simulink model "Big_system"  (R2025b)
settings: Solver=ode8  StartTime=0.0  StopTime=60*80  FixedStep=1  RelTol=1e-3
model workspace (MAT data in the model file):
  Sig = Simulink.Signal
  Sig.Dimensions = -1
  Sig.DimensionsMode = 'auto'
  Sig.Complexity = 'auto'
  Sig.SampleTime = -1
  Sig.SamplingMode = 'auto'
  Sig.DataType = 'auto'
settings Model: Creator=Soere  LastModifiedBy=klump
settings DebuggingCC: UnderSpecifiedDimensionMsg=warning

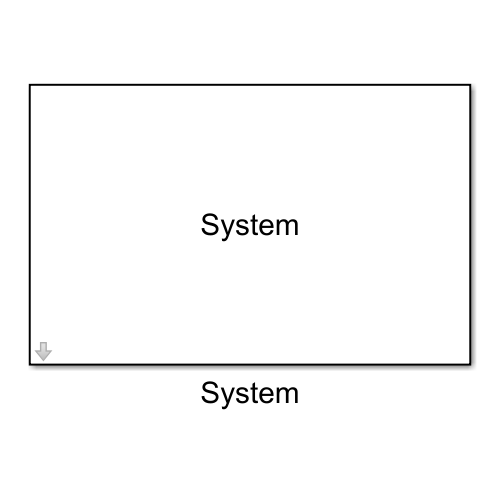
[thumbnail: Simulink's stored preview of the top-level diagram]
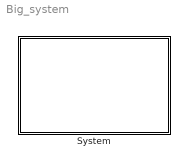
== system Big_system ==
  System : Subsystem  mask{RainSmallStart=(60*20)/4 * 0, RainSmall=5/5, RainSmallDur=60*20, RainBig=20/5, RainBigDur=(60*20)/4, ProcessingRate=9, flip_order=off, EnableBurst_1=on, EnableBurst_4=off, EnableBurst_2=off, EnableBurst_5=on, EnableBurst_3=off, EnableBurst_6=off}
      mask prompts: RainSmallStart "Start of rain:"; RainSmall "Normal rainfall (liters/minute):"; RainSmallDur "Normal Rainfall Duration:"; RainBig "Cloudburst (liters/minute):"; RainBigDur "Cloudburst duration (sec):"; ProcessingRate "Processing rate:"; flip_order "Flip order"; EnableBurst_1 "Enable cloud burst 1"; EnableBurst_4 "Enable cloud burst 4"; EnableBurst_2 "Enable cloud burst 2"; EnableBurst_5 "Enable cloud burst 5"; EnableBurst_3 "Enable cloud burst 3"; EnableBurst_6 "Enable cloud burst 6"
      mask TypeOptions flip_order: Final/flip_order | Subsystem 1/flip_order | Subsystem 1/flip_order_2 | Subsystem 2/flip_order | Subsystem 2/flip_order_2 | Subsystem 3/flip_order | Subsystem 4/flip_order | Subsystem 4/flip_order_2 | Subsystem 5/flip_order | Subsystem 6/flip_order | Subsystem 6/flip_order_2
      mask TypeOptions EnableBurst_1: Subsystem 1/EnableBurst
      mask TypeOptions EnableBurst_4: Subsystem 4/EnableBurst
      mask TypeOptions EnableBurst_2: Subsystem 2/EnableBurst
      mask TypeOptions EnableBurst_5: Subsystem 5/EnableBurst
      mask TypeOptions EnableBurst_3: Subsystem 3/EnableBurst
      mask TypeOptions EnableBurst_6: Final/EnableBurst | Subsystem 6/EnableBurst
      mask DialogControl Container3 Prompt: Enable cloudbursts:
      mask Display: disp('System');

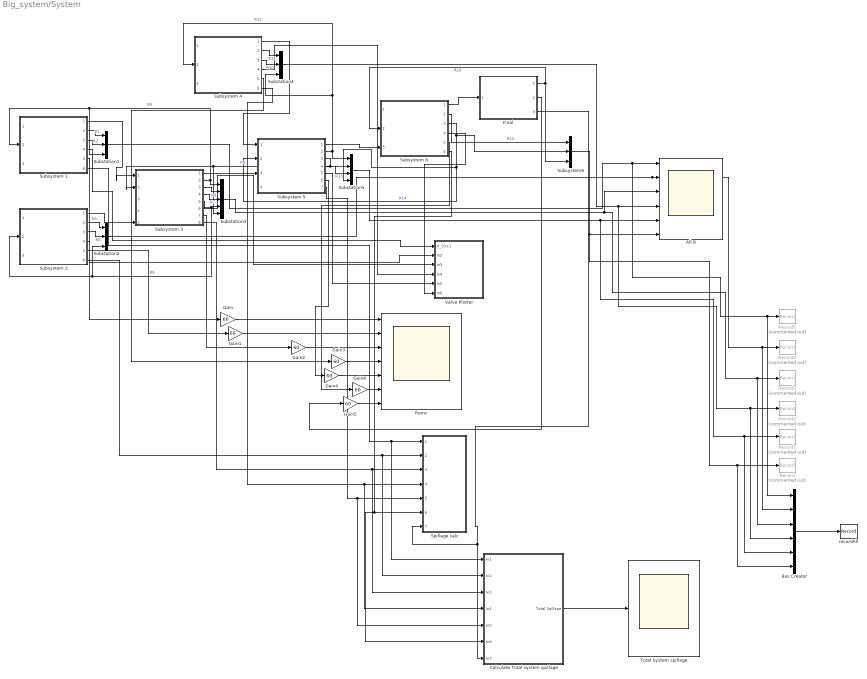
== system Big_system/System ==
  All R : Scope  NumInputPorts=6
      settings: ActiveDisplayString=6  Title=Subsystem 6  ActiveDisplayYMinimum=-5  ActiveDisplayYMaximum=30  YLabel=Remaining capacity (liters)  DataLoggingVariableName=ScopeData34
  Bus Creator : BusCreator  Inputs=6
  Calculate Total system spillage : Subsystem
  Final : Subsystem  ReferencedSubsystem=Subsystem_last  Waterlevel_1=0  proces=ProcessingRate  Diameter=23.3  Max_cap_1=510-150  Duration=RainSmallDur  Flowrate=RainSmall  BurstStart=RainBigDur  BurstFlow=RainBig  BurstDur=RainBigDur  rain_start=RainSmallStart  station_order=4  flip_order=off  RainSwitch_S1=on  EnableBurst=off
  Gain{,1..6} (7 alike) : Gain  Gain=60
  Rains : Scope  NumInputPorts=7
      settings: ActiveDisplayString=6  Title=Subsystem 6  ActiveDisplayYMinimum=-0.1  ActiveDisplayYMaximum=4.1  YLabel=Flowrate (l/min)  DataLoggingVariableName=ScopeData16
  Record : Record  Commented=on  NumPorts=1.0  Filename=C:\Users\klump\OneDrive - Aalborg Universitet\P8\Project\Simulation\plots\substation6.mldatx  RecordToFile=on  FileSettingsInternal="{\"entries\":[{\"content\":{\"excelSettings\":{\"content\":{},\"type\":\"Streamout.ExcelSettings\"},\"parquetSettings\":{\"content\":{},\"type\":\"Streamout.ParquetSettings\"}},\"type\":\"Streamout.FileSettingStorage\",\"uuid\":\"\"}],\"packageUris\":[\"http:\\/\\/schema.mathworks.com\\/mf0\\/streamout_blocks\\/R2020a\"],\"version\":\"1.0\"}"  FrameSettings=0  Layout=[1 1]  SignalsInternal="{\"entries\":[{\"content\":{\"signals\":[{\"content\":{\"blockPath\":[],\"dimensions\":[1],\"domain\":\"\",\"hasChildren\":true,\"lineColor\":\"#ff6929\",\"lineWidth\":2,\"port\":1,\"signalID\":1,\"signalName\":\"Subsystem6\"},\"type\":\"RecordBlkView.Signal\",\"uuid\":\"\"},{\"content\":{\"blockPath\":[],\"dimensions\":[1],\"domain\":\"\",\"leafPath\":\"Subsystem6.R15\",\"lineColor\":\"#22b573\",\"lineWidth\":2,\"parentID\":1,\"port\":1,\"signalID\":2,\"signalName\":\"Subsystem6.R15\"},\"type\":\"RecordBlkView.Signal\",\"uuid\":\"\"},{\"content\":{\"blockPath\":[],\"dimensions\":[1],\"domain\":\"\",\"leafPath\":\"Subsystem6.R14\",\"lineColor\":\"#0072bd\",\"lineWidth\":2,\"parentID\":1,\"port\":1,\"signalID\":3,\"signalName\":\"Subsystem6.R14\"},\"type\":\"RecordBlkView.Signal\",\"uuid\":\"\"},{\"content\":{\"blockPath\":[],\"dimensions\":[1],\"domain\":\"\",\"leafPath\":\"Subsystem6.R16\",\"lineColor\":\"#d95319\",\"lineWidth\":2,\"parentID\":1,\"port\":1,\"signalID\":4,\"signalName\":\"Subsystem6.R16\"},\"type\":\"RecordBlkView.Signal\",\"uuid\":\"\"}]},\"type\":\"RecordBlkView.InputSignals\",\"uuid\":\"\"}],\"packageUris\":[\"http:\\/\\/schema.mathworks.com\\/mf0\\/streamout_blocks\\/R2020a\"],\"version\":\"1.0\"}"
  Record1 : Record  Commented=on  NumPorts=1.0  Filename=C:\Users\klump\OneDrive - Aalborg Universitet\P8\Project\Simulation\plots\substation5.mldatx  RecordToFile=on  FileSettingsInternal="{\"entries\":[{\"content\":{\"excelSettings\":{\"content\":{},\"type\":\"Streamout.ExcelSettings\"},\"parquetSettings\":{\"content\":{},\"type\":\"Streamout.ParquetSettings\"}},\"type\":\"Streamout.FileSettingStorage\",\"uuid\":\"\"}],\"packageUris\":[\"http:\\/\\/schema.mathworks.com\\/mf0\\/streamout_blocks\\/R2020a\"],\"version\":\"1.0\"}"  FrameSettings=0  Layout=[1 1]  SignalsInternal="{\"entries\":[{\"content\":{\"signals\":[{\"content\":{\"blockPath\":[],\"dimensions\":[1],\"domain\":\"\",\"hasChildren\":true,\"lineColor\":\"#fe330a\",\"lineWidth\":2,\"port\":1,\"signalID\":1,\"signalName\":\"Substation5\"},\"type\":\"RecordBlkView.Signal\",\"uuid\":\"\"},{\"content\":{\"blockPath\":[],\"dimensions\":[1],\"domain\":\"\",\"leafPath\":\"Substation5.R12\",\"lineColor\":\"#7e2f8e\",\"lineWidth\":2,\"parentID\":1,\"port\":1,\"signalID\":2,\"signalName\":\"Substation5.R12\"},\"type\":\"RecordBlkView.Signal\",\"uuid\":\"\"},{\"content\":{\"blockPath\":[],\"dimensions\":[1],\"domain\":\"\",\"leafPath\":\"Substation5.R9\",\"lineColor\":\"#77ac30\",\"lineWidth\":2,\"parentID\":1,\"port\":1,\"signalID\":3,\"signalName\":\"Substation5.R9\"},\"type\":\"RecordBlkView.Signal\",\"uuid\":\"\"},{\"content\":{\"blockPath\":[],\"dimensions\":[1],\"domain\":\"\",\"leafPath\":\"Substation5.R13\",\"lineColor\":\"#4dbeee\",\"lineWidth\":2,\"parentID\":1,\"port\":1,\"signalID\":4,\"signalName\":\"Substation5.R13\"},\"type\":\"RecordBlkView.Signal\",\"uuid\":\"\"},{\"content\":{\"blockPath\":[],\"dimensions\":[1],\"domain\":\"\",\"leafPath\":\"Substation5.R14\",\"lineColor\":\"#a2142f\",\"lineWidth\":2,\"parentID\":1,\"port\":1,\"signalID\":5,\"signalName\":\"Substation5.R14\"},\"type\":\"RecordBlkView.Signal\",\"uuid\":\"\"}]},\"type\":\"RecordBlkView.InputSignals\",\"uuid\":\"\"}],\"packageUris\":[\"http:\\/\\/schema.mathworks.com\\/mf0\\/streamout_blocks\\/R2020a\"],\"version\":\"1.0\"}"
  Record2 : Record  Commented=on  NumPorts=1.0  Filename=C:\Users\klump\OneDrive - Aalborg Universitet\P8\Project\Simulation\plots\substation4.mldatx  RecordToFile=on  FileSettingsInternal="{\"entries\":[{\"content\":{\"excelSettings\":{\"content\":{},\"type\":\"Streamout.ExcelSettings\"},\"parquetSettings\":{\"content\":{},\"type\":\"Streamout.ParquetSettings\"}},\"type\":\"Streamout.FileSettingStorage\",\"uuid\":\"\"}],\"packageUris\":[\"http:\\/\\/schema.mathworks.com\\/mf0\\/streamout_blocks\\/R2020a\"],\"version\":\"1.0\"}"  FrameSettings=0  Layout=[1 1]  SignalsInternal="{\"entries\":[{\"content\":{\"signals\":[{\"content\":{\"blockPath\":[],\"dimensions\":[1],\"domain\":\"\",\"hasChildren\":true,\"lineColor\":\"#7e2f8e\",\"lineWidth\":2,\"port\":1,\"signalID\":1,\"signalName\":\"Substation4\"},\"type\":\"RecordBlkView.Signal\",\"uuid\":\"\"},{\"content\":{\"blockPath\":[],\"dimensions\":[1],\"domain\":\"\",\"leafPath\":\"Substation4.R11\",\"lineColor\":\"#ff6929\",\"lineWidth\":2,\"parentID\":1,\"port\":1,\"signalID\":2,\"signalName\":\"Substation4.R11\"},\"type\":\"RecordBlkView.Signal\",\"uuid\":\"\"},{\"content\":{\"blockPath\":[],\"dimensions\":[1],\"domain\":\"\",\"leafPath\":\"Substation4.R10\",\"lineColor\":\"#b746ff\",\"lineWidth\":2,\"parentID\":1,\"port\":1,\"signalID\":3,\"signalName\":\"Substation4.R10\"},\"type\":\"RecordBlkView.Signal\",\"uuid\":\"\"},{\"content\":{\"blockPath\":[],\"dimensions\":[1],\"domain\":\"\",\"leafPath\":\"Substation4.R12\",\"lineColor\":\"#64d413\",\"lineWidth\":2,\"parentID\":1,\"port\":1,\"signalID\":4,\"signalName\":\"Substation4.R12\"},\"type\":\"RecordBlkView.Signal\",\"uuid\":\"\"}]},\"type\":\"RecordBlkView.InputSignals\",\"uuid\":\"\"}],\"packageUris\":[\"http:\\/\\/schema.mathworks.com\\/mf0\\/streamout_blocks\\/R2020a\"],\"version\":\"1.0\"}"
  Record3 : Record  Commented=on  NumPorts=1.0  Filename=C:\Users\klump\OneDrive - Aalborg Universitet\P8\Project\Simulation\plots\substation3.mldatx  RecordToFile=on  FileSettingsInternal="{\"entries\":[{\"content\":{\"excelSettings\":{\"content\":{},\"type\":\"Streamout.ExcelSettings\"},\"parquetSettings\":{\"content\":{},\"type\":\"Streamout.ParquetSettings\"}},\"type\":\"Streamout.FileSettingStorage\",\"uuid\":\"\"}],\"packageUris\":[\"http:\\/\\/schema.mathworks.com\\/mf0\\/streamout_blocks\\/R2020a\"],\"version\":\"1.0\"}"  FrameSettings=0  Layout=[1 1]  SignalsInternal="{\"entries\":[{\"content\":{\"signals\":[{\"content\":{\"blockPath\":[],\"dimensions\":[1],\"domain\":\"\",\"hasChildren\":true,\"lineColor\":\"#139fff\",\"lineWidth\":2,\"port\":1,\"signalID\":1,\"signalName\":\"Substation3\"},\"type\":\"RecordBlkView.Signal\",\"uuid\":\"\"},{\"content\":{\"blockPath\":[],\"dimensions\":[1],\"domain\":\"\",\"leafPath\":\"Substation3.R5\",\"lineColor\":\"#fe330a\",\"lineWidth\":2,\"parentID\":1,\"port\":1,\"signalID\":2,\"signalName\":\"Substation3.R5\"},\"type\":\"RecordBlkView.Signal\",\"uuid\":\"\"},{\"content\":{\"blockPath\":[],\"dimensions\":[1],\"domain\":\"\",\"leafPath\":\"Substation3.R6\",\"lineColor\":\"#22b573\",\"lineWidth\":2,\"parentID\":1,\"port\":1,\"signalID\":3,\"signalName\":\"Substation3.R6\"},\"type\":\"RecordBlkView.Signal\",\"uuid\":\"\"},{\"content\":{\"blockPath\":[],\"dimensions\":[1],\"domain\":\"\",\"leafPath\":\"Substation3.R7\",\"lineColor\":\"#0072bd\",\"lineWidth\":2,\"parentID\":1,\"port\":1,\"signalID\":4,\"signalName\":\"Substation3.R7\"},\"type\":\"RecordBlkView.Signal\",\"uuid\":\"\"},{\"content\":{\"blockPath\":[],\"dimensions\":[1],\"domain\":\"\",\"leafPath\":\"Substation3.R8\",\"lineColor\":\"#d95319\",\"lineWidth\":2,\"parentID\":1,\"port\":1,\"signalID\":5,\"signalName\":\"Substation3.R8\"},\"type\":\"RecordBlkView.Signal\",\"uuid\":\"\"},{\"content\":{\"blockPath\":[],\"dimensions\":[1],\"domain\":\"\",\"leafPath\":\"Substation3.R9\",\"lineColor\":\"#edb120\",\"lineWidth\":2,\"parentID\":1,\"port\":1,\"signalID\":6,\"signalName\":\"Substation3.R9\"},\"type\":\"RecordBlkView.Signal\",\"uuid\":\"\"}]},\"type\":\"RecordBlkView.InputSignals\",\"uuid\":\"\"}],\"packageUris\":[\"http:\\/\\/schema.mathworks.com\\/mf0\\/streamout_blocks\\/R2020a\"],\"version\":\"1.0\"}"
  Record4 : Record  Commented=on  NumPorts=1.0  Filename=C:\Users\klump\OneDrive - Aalborg Universitet\P8\Project\Simulation\plots\substation2.mldatx  RecordToFile=on  FileSettingsInternal="{\"entries\":[{\"content\":{\"excelSettings\":{\"content\":{},\"type\":\"Streamout.ExcelSettings\"},\"parquetSettings\":{\"content\":{},\"type\":\"Streamout.ParquetSettings\"}},\"type\":\"Streamout.FileSettingStorage\",\"uuid\":\"\"}],\"packageUris\":[\"http:\\/\\/schema.mathworks.com\\/mf0\\/streamout_blocks\\/R2020a\"],\"version\":\"1.0\"}"  FrameSettings=0  Layout=[1 1]  SignalsInternal="{\"entries\":[{\"content\":{\"signals\":[{\"content\":{\"blockPath\":[],\"dimensions\":[1],\"domain\":\"\",\"hasChildren\":true,\"lineColor\":\"#22b573\",\"lineWidth\":2,\"port\":1,\"signalID\":1,\"signalName\":\"Substation2\"},\"type\":\"RecordBlkView.Signal\",\"uuid\":\"\"},{\"content\":{\"blockPath\":[],\"dimensions\":[1],\"domain\":\"\",\"leafPath\":\"Substation2.R3\",\"lineColor\":\"#77ac30\",\"lineWidth\":2,\"parentID\":1,\"port\":1,\"signalID\":2,\"signalName\":\"Substation2.R3\"},\"type\":\"RecordBlkView.Signal\",\"uuid\":\"\"},{\"content\":{\"blockPath\":[],\"dimensions\":[1],\"domain\":\"\",\"leafPath\":\"Substation2.R4\",\"lineColor\":\"#4dbeee\",\"lineWidth\":2,\"parentID\":1,\"port\":1,\"signalID\":3,\"signalName\":\"Substation2.R4\"},\"type\":\"RecordBlkView.Signal\",\"uuid\":\"\"},{\"content\":{\"blockPath\":[],\"dimensions\":[1],\"domain\":\"\",\"leafPath\":\"Substation2.R8\",\"lineColor\":\"#a2142f\",\"lineWidth\":2,\"parentID\":1,\"port\":1,\"signalID\":4,\"signalName\":\"Substation2.R8\"},\"type\":\"RecordBlkView.Signal\",\"uuid\":\"\"}]},\"type\":\"RecordBlkView.InputSignals\",\"uuid\":\"\"}],\"packageUris\":[\"http:\\/\\/schema.mathworks.com\\/mf0\\/streamout_blocks\\/R2020a\"],\"version\":\"1.0\"}"
  Record5 : Record  Commented=on  NumPorts=1.0  Filename=C:\Users\klump\OneDrive - Aalborg Universitet\P8\Project\Simulation\plots\substation1.mldatx  RecordToFile=on  FileSettingsInternal="{\"entries\":[{\"content\":{\"excelSettings\":{\"content\":{},\"type\":\"Streamout.ExcelSettings\"},\"parquetSettings\":{\"content\":{},\"type\":\"Streamout.ParquetSettings\"}},\"type\":\"Streamout.FileSettingStorage\",\"uuid\":\"\"}],\"packageUris\":[\"http:\\/\\/schema.mathworks.com\\/mf0\\/streamout_blocks\\/R2020a\"],\"version\":\"1.0\"}"  FrameSettings=0  Layout=[1 1]  SignalsInternal="{\"entries\":[{\"content\":{\"signals\":[{\"content\":{\"blockPath\":[],\"dimensions\":[1],\"domain\":\"\",\"hasChildren\":true,\"lineColor\":\"#7e2f8e\",\"lineWidth\":2,\"port\":1,\"signalID\":1,\"signalName\":\"Substation1\"},\"type\":\"RecordBlkView.Signal\",\"uuid\":\"\"},{\"content\":{\"blockPath\":[],\"dimensions\":[1],\"domain\":\"\",\"leafPath\":\"Substation1.R1\",\"lineColor\":\"#ff6929\",\"lineWidth\":2,\"parentID\":1,\"port\":1,\"signalID\":2,\"signalName\":\"Substation1.R1\"},\"type\":\"RecordBlkView.Signal\",\"uuid\":\"\"},{\"content\":{\"blockPath\":[],\"dimensions\":[1],\"domain\":\"\",\"leafPath\":\"Substation1.R2\",\"lineColor\":\"#b746ff\",\"lineWidth\":2,\"parentID\":1,\"port\":1,\"signalID\":3,\"signalName\":\"Substation1.R2\"},\"type\":\"RecordBlkView.Signal\",\"uuid\":\"\"},{\"content\":{\"blockPath\":[],\"dimensions\":[1],\"domain\":\"\",\"leafPath\":\"Substation1.R5\",\"lineColor\":\"#64d413\",\"lineWidth\":2,\"parentID\":1,\"port\":1,\"signalID\":4,\"signalName\":\"Substation1.R5\"},\"type\":\"RecordBlkView.Signal\",\"uuid\":\"\"}]},\"type\":\"RecordBlkView.InputSignals\",\"uuid\":\"\"}],\"packageUris\":[\"http:\\/\\/schema.mathworks.com\\/mf0\\/streamout_blocks\\/R2020a\"],\"version\":\"1.0\"}"
  Spillage calc : Subsystem
  Substation1 : BusCreator  Inputs=3
  Substation2 : BusCreator  Inputs=3
  Substation3 : BusCreator  Inputs=5
  Substation4 : BusCreator  Inputs=3
  Substation5 : BusCreator  Inputs=4
  Subsystem 1 : Subsystem  ReferencedSubsystem=Subsystem_2S  station_order=1  RainSwitch_S1=on  flip_order=off  Waterlevel_1=0  Height=1  K=7.77*1e-5  Max_cap_1=703-150  Diameter=24.5  BurstStart=RainBigDur  BurstFlow=RainBig  BurstDur=RainBigDur  rain_start=RainSmallStart  Duration_S1=RainSmallDur  Flowrate_S1=RainSmall  A=0.0117  B=0.1252  Parameter37=0  Parameter35=0  Parameter36=0  Parameter38=0  Parameter39=0  Waterlevel_2=0  Height_2=1  Max_cap_2=695-150  Diameter_2=23.3  K_2=7.32*1e-5  A_2=0.0118  B_2=0.1206  Duration_S2=RainSmallDur  Flowrate_S2=RainSmall  BurstStart_2=RainBigDur  BurstFlow_2=RainBig  BurstDur_2=RainBigDur  rain_start_2=RainSmallStart  station_order_2=1  flip_order_2=off  RainSwitch_S2=on  DelayLength=0  EnableBurst=on
  Subsystem 2 : Subsystem  ReferencedSubsystem=Subsystem_2S  station_order=1  RainSwitch_S1=on  flip_order=off  Waterlevel_1=0  Height=1  K=7.77*1e-5  Max_cap_1=703-150  Diameter=24.5  BurstStart=RainBigDur*1  BurstFlow=RainBig  BurstDur=RainBigDur  rain_start=RainSmallStart  Duration_S1=RainSmallDur  Flowrate_S1=RainSmall  A=0.0117  B=0.1252  Parameter37=0  Parameter35=0  Parameter36=0  Parameter38=0  Parameter39=0  Waterlevel_2=0  Height_2=1  Max_cap_2=695-150  Diameter_2=23.3  K_2=7.32*1e-5  A_2=0.0118  B_2=0.1206  Duration_S2=RainSmallDur  Flowrate_S2=RainSmall  BurstStart_2=RainBigDur*1  BurstFlow_2=RainBig  BurstDur_2=RainBigDur  rain_start_2=RainSmallStart  station_order_2=1  flip_order_2=off  RainSwitch_S2=on  DelayLength=0  EnableBurst=off
  Subsystem 3 : Subsystem  ReferencedSubsystem=Subsystem_4S  Waterlevel_1=0  Height=1  Max_cap_1=703-150  Diameter=24.5  K=7.77*1e-5  A=0.0117  B=0.1252  Duration_S1=RainSmallDur  Flowrate_S1=RainSmall  BurstStart=RainBigDur  BurstFlow=RainBig  BurstDur=RainBigDur  RainSwitch_S1=on  Waterlevel_2=0  Height_2=1  Max_cap_2=695-150  Diameter_2=23.3  K_2=7.32*1e-5  A_2=0.0118  B_2=0.1206  Duration_2=RainSmallDur  Flowrate_2=RainSmall  BurstStart_2=RainBigDur  BurstFlow_2=RainBig  BurstDur_2=RainBigDur  RainSwitch_S2=on  InitialCondition=0  Height_3=1  Max_cap_3=703-150  Diameter_3=24.5  K_3=7.77*1e-5  A_3=0.0117  B_3=0.1252  Duration_3=RainSmallDur  Flowrate_3=RainSmall  BurstStart_3=RainBigDur  BurstFlow_3=RainBig  BurstDur_3=RainBigDur  RainSwitch_S3=on  InitialCondition_4=0  Height_4=1  Max_cap_4=695-150  Diameter_4=23.3  K_4=7.32*1e-5  A_4=0.0118  B_4=0.1206  Duration_4=RainSmallDur  Flowrate_4=RainSmall  BurstStart_4=RainBigDur  BurstFlow_4=RainBig  BurstDur_4=RainBigDur  RainSwitch_S4=on  DelayLength=0  rain_start=RainSmallStart  station_order=2  flip_order=off  EnableBurst=off
  Subsystem 4 : Subsystem  ReferencedSubsystem=Subsystem_2S  station_order=3  RainSwitch_S1=on  flip_order=off  Waterlevel_1=0  Height=1  K=7.77*1e-5  Max_cap_1=703-150  Diameter=24.5  BurstStart=RainBigDur  BurstFlow=RainBig  BurstDur=RainBigDur  rain_start=RainSmallStart  Duration_S1=RainSmallDur  Flowrate_S1=RainSmall  A=0.0117  B=0.1252  Parameter37=0  Parameter35=0  Parameter36=0  Parameter38=0  Parameter39=0  Waterlevel_2=0  Height_2=1  Max_cap_2=695-150  Diameter_2=23.3  K_2=7.32*1e-5  A_2=0.0118  B_2=0.1206  Duration_S2=RainSmallDur  Flowrate_S2=RainSmall  BurstStart_2=RainBigDur  BurstFlow_2=RainBig  BurstDur_2=RainBigDur  rain_start_2=RainSmallStart  station_order_2=3  flip_order_2=off  RainSwitch_S2=on  DelayLength=0  EnableBurst=off
  Subsystem 5 : Subsystem  ReferencedSubsystem=Subsystem_3S  Waterlevel_1=0  Height=1  Max_cap_1=703-150  Diameter=24.5  K=7.77*1e-5  A=0.0117  B=0.1252  Duration_S1=RainSmallDur  Flowrate_S1=RainSmall  BurstStart=RainBigDur  BurstFlow=RainBig  BurstDur=RainBigDur  RainSwitch_S1=on  Waterlevel_2=0  Height_2=1  Max_cap_2=695-150  Diameter_2=23.3  K_2=7.32*1e-5  A_2=0.0118  B_2=0.1206  Duration_2=RainSmallDur  Flowrate_2=RainSmall  BurstStart_2=RainBigDur  BurstFlow_2=RainBig  BurstDur_2=RainBigDur  RainSwitch_S2=on  InitialCondition=0  Height_3=1  Max_cap_3=703-150  Diameter_3=24.5  K_3=7.77*1e-5  A_3=0.0117  B_3=0.1252  Duration_3=RainSmallDur  Flowrate_3=RainSmall  BurstStart_3=RainBigDur  BurstFlow_3=RainBig  BurstDur_3=RainBigDur  RainSwitch_S3=on  DelayLength=0  rain_start=RainSmallStart  station_order=3  flip_order=off  EnableBurst=on
  Subsystem 6 : Subsystem  ReferencedSubsystem=Subsystem_2S  station_order=4  RainSwitch_S1=on  flip_order=off  Waterlevel_1=0  Height=1  K=7.77*1e-5  Max_cap_1=703-150  Diameter=24.5  BurstStart=RainBigDur  BurstFlow=RainBig  BurstDur=RainBigDur*1  rain_start=RainSmallStart  Duration_S1=RainSmallDur  Flowrate_S1=RainSmall  A=0.0117  B=0.1252  Parameter37=0  Parameter35=0  Parameter36=0  Parameter38=0  Parameter39=0  Waterlevel_2=0  Height_2=1  Max_cap_2=695-150  Diameter_2=23.3  K_2=7.32*1e-5  A_2=0.0118  B_2=0.1206  Duration_S2=RainSmallDur  Flowrate_S2=RainSmall  BurstStart_2=RainBigDur  BurstFlow_2=RainBig  BurstDur_2=RainBigDur  rain_start_2=RainSmallStart  station_order_2=4  flip_order_2=off  RainSwitch_S2=on  DelayLength=0  EnableBurst=off
  Subsystem6 : BusCreator  Inputs=3
  Total System spillage : Scope
      settings: ActiveDisplayYMinimum=-5  ActiveDisplayYMaximum=60  YLabel=Total spillage (liters)  DataLoggingVariableName=ScopeData89
  Valve Plotter : Subsystem
  recordAll : Record  NumPorts=1.0  Filename=C:\Users\klump\OneDrive - Aalborg Universitet\P8\Project\Simulation\plots\substation_all.mldatx  RecordToFile=on  FileSettingsInternal="{\"entries\":[{\"content\":{\"excelSettings\":{\"content\":{},\"type\":\"Streamout.ExcelSettings\"},\"parquetSettings\":{\"content\":{},\"type\":\"Streamout.ParquetSettings\"}},\"type\":\"Streamout.FileSettingStorage\",\"uuid\":\"\"}],\"packageUris\":[\"http:\\/\\/schema.mathworks.com\\/mf0\\/streamout_blocks\\/R2020a\"],\"version\":\"1.0\"}"  FrameSettings=0  Layout=[2 3]  SignalsInternal="{\"entries\":[{\"content\":{\"signals\":[{\"content\":{\"blockPath\":[],\"dimensions\":[1],\"domain\":\"\",\"hasChildren\":true,\"lineColor\":\"#22b573\",\"lineWidth\":2,\"port\":1,\"sid\":[\"\"],\"signalID\":1,\"signalName\":\"Bus\\nCreator\"},\"type\":\"RecordBlkView.Signal\",\"uuid\":\"\"},{\"content\":{\"blockPath\":[],\"dimensions\":[1],\"domain\":\"\",\"hasChildren\":true,\"lineColor\":\"#0072bd\",\"lineWidth\":2,\"parentID\":1,\"port\":1,\"sid\":[\"\"],\"signalID\":2,\"signalName\":\"signal1\"},\"type\":\"RecordBlkView.Signal\",\"uuid\":\"\"},{\"content\":{\"blockPath\":[],\"dimensions\":[1],\"domain\":\"\",\"leafPath\":\"Bus\\nCreator.signal1.R1\",\"lineColor\":\"#22b573\",\"lineWidth\":2,\"parentID\":2,\"plots\":[ 1 ],\"port\":1,\"sid\":[\"\"],\"signalID\":3,\"signalName\":\"Bus\\nCreator.signal1.R1\"},\"type\":\"RecordBlkView.Signal\",\"uuid\":\"\"},{\"content\":{\"blockPath\":[],\"dimensions\":[1],\"domain\":\"\",\"leafPath\":\"Bus\\nCreator.signal1.R2\",\"lineColor\":\"#0072bd\",\"lineWidth\":2,\"parentID\":2,\"plots\":[ 1 ],\"port\":1,\"sid\":[\"\"],\"signalID\":4,\"signalName\":\"Bus\\nCreator.signal1.R2\"},\"type\":\"RecordBlkView.Signal\",\"uuid\":\"\"},{\"content\":{\"blockPath\":[],\"dimensions\":[1],\"domain\":\"\",\"leafPath\":\"Bus\\nCreator.signal1.R5\",\"lineColor\":\"#d95319\",\"lineWidth\":2,\"parentID\":2,\"plots\":[ 1 ],\"port\":1,\"sid\":[\"\"],\"signalID\":5,\"signalName\":\"Bus\\nCreator.signal1.R5\"},\"type\":\"RecordBlkView.Signal\",\"uuid\":\"\"},{\"content\":{\"blockPath\":[],\"dimensions\":[1],\"domain\":\"\",\"hasChildren\":true,\"lineColor\":\"#77ac30\",\"lineWidth\":2,\"parentID\":1,\"port\":1,\"sid\":[\"\"],\"signalID\":6,\"signalName\":\"signal2\"},\"type\":\"RecordBlkView.Signal\",\"uuid\":\"\"},{\"content\":{\"blockPath\":[],\"dimensions\":[1],\"domain\":\"\",\"leafPath\":\"Bus\\nCreator.signal2.R3\",\"lineColor\":\"#7e2f8e\",\"lineWidth\":2,\"parentID\":6,\"plots\":[ 2 ],\"port\":1,\"sid\":[\"\"],\"signalID\":7,\"signalName\":\"Bus\\nCreator.signal2.R3\"},\"type\":\"RecordBlkView.Signal\",\"uuid\":\"\"},{\"content\":{\"blockPath\":[],\"dimensions\":[1],\"domain\":\"\",\"leafPath\":\"Bus\\nCreator.signal2.R4\",\"lineColor\":\"#77ac30\",\"lineWidth\":2,\"parentID\":6,\"plots\":[ 2 ],\"port\":1,\"sid\":[\"\"],\"signalID\":8,\"signalName\":\"Bus\\nCreator.signal2.R4\"},\"type\":\"RecordBlkView.Signal\",\"uuid\":\"\"},{\"content\":{\"blockPath\":[],\"dimensions\":[1],\"domain\":\"\",\"leafPath\":\"Bus\\nCreator.signal2.R8\",\"lineColor\":\"#4dbeee\",\"lineWidth\":2,\"parentID\":6,\"plots\":[ 2 ],\"port\":1,\"sid\":[\"\"],\"signalID\":9,\"signalName\":\"Bus\\nCreator.signal2.R8\"},\"type\":\"RecordBlkView.Signal\",\"uuid\":\"\"},{\"content\":{\"blockPath\":[],\"dimensions\":[1],\"domain\":\"\",\"hasChildren\":true,\"lineColor\":\"#ff6929\",\"lineWidth\":2,\"parentID\":1,\"port\":1,\"sid\":[\"\"],\"signalID\":10,\"signalName\":\"signal3\"},\"type\":\"RecordBlkView.Signal\",\"uuid\":\"\"},{\"content\":{\"blockPath\":[],\"dimensions\":[1],\"domain\":\"\",\"leafPath\":\"Bus\\nCreator.signal3.R5\",\"lineColor\":\"#139fff\",\"lineWidth\":2,\"parentID\":10,\"plots\":[ 9 ],\"port\":1,\"sid\":[\"\"],\"signalID\":11,\"signalName\":\"Bus\\nCreator.signal3.R5\"},\"type\":\"RecordBlkView.Signal\",\"uuid\":\"\"},{\"content\":{\"blockPath\":[],\"dimensions\":[1],\"domain\":\"\",\"leafPath\":\"Bus\\nCreator.signal3.R6\",\"lineColor\":\"#ff6929\",\"lineWidth\":2,\"parentID\":10,\"plots\":[ 9 ],\"port\":1,\"sid\":[\"\"],\"signalID\":12,\"signalName\":\"Bus\\nCreator.signal3.R6\"},\"type\":\"RecordBlkView.Signal\",\"uuid\":\"\"},{\"content\":{\"blockPath\":[],\"dimensions\":[1],\"domain\":\"\",\"leafPath\":\"Bus\\nCreator.signal3.R7\",\"lineColor\":\"#b746ff\",\"lineWidth\":2,\"parentID\":10,\"plots\":[ 9 ],\"port\":1,\"sid\":[\"\"],\"signalID\":13,\"signalName\":\"Bus\\nCreator.signal3.R7\"},\"type\":\"RecordBlkView.Signal\",\"uuid\":\"\"},{\"content\":{\"blockPath\":[],\"dimensions\":[1],\"domain\":\"\",\"leafPath\":\"Bus\\nCreator.signal3.R8\",\"lineColor\":\"#64d413\",\"lineWidth\":2,\"parentID\":10,\"plots\":[ 9 ],\"port\":1,\"sid\":[\"\"],\"signalID\":14,\"signalName\":\"Bus\\nCreator.signal3.R8\"},\"type\":\"RecordBlkView.Signal\",\"uuid\":\"\"},{\"content\":{\"blockPath\":[],\"dimensions\":[1],\"domain\":\"\",\"leafPath\":\"Bus\\nCreator.signal3.R9\",\"lineColor\":\"#ff13a6\",\"lineWidth\":2,\"parentID\":10,\"plots\":[ 9 ],\"port\":1,\"sid\":[\"\"],\"signalID\":15,\"signalName\":\"Bus\\nCreator.signal3.R9\"},\"type\":\"RecordBlkView.Signal\",\"uuid\":\"\"},{\"content\":{\"blockPath\":[],\"dimensions\":[1],\"domain\":\"\",\"hasChildren\":true,\"lineColor\":\"#0072bd\",\"lineWidth\":2,\"parentID\":1,\"port\":1,\"sid\":[\"\"],\"signalID\":16,\"signalName\":\"signal4\"},\"type\":\"RecordBlkView.Signal\",\"uuid\":\"\"},{\"content\":{\"blockPath\":[],\"dimensions\":[1],\"domain\":\"\",\"leafPath\":\"Bus\\nCreator.signal4.R11\",\"lineColor\":\"#22b573\",\"lineWidth\":2,\"parentID\":16,\"plots\":[ 10 ],\"port\":1,\"sid\":[\"\"],\"signalID\":17,\"signalName\":\"Bus\\nCreator.signal4.R11\"},\"type\":\"RecordBlkView.Signal\",\"uuid\":\"\"},{\"content\":{\"blockPath\":[],\"dimensions\":[1],\"domain\":\"\",\"leafPath\":\"Bus\\nCreator.signal4.R10\",\"lineColor\":\"#0072bd\",\"lineWidth\":2,\"parentID\":16,\"plots\":[ 10 ],\"port\":1,\"sid\":[\"\"],\"signalID\":18,\"signalName\":\"Bus\\nCreator.signal4.R10\"},\"type\":\"RecordBlkView.Signal\",\"uuid\":\"\"},{\"content\":{\"blockPath\":[],\"dimensions\":[1],\"domain\":\"\",\"leafPath\":\"Bus\\nCreator.signal4.R12\",\"lineColor\":\"#d95319\",\"lineWidth\":2,\"parentID\":16,\"plots\":[ 10 ],\"port\":1,\"sid\":[\"\"],\"signalID\":19,\"signalName\":\"Bus\\nCreator.signal4.R12\"},\"type\":\"RecordBlkView.Signal\",\"uuid\":\"\"},{\"content\":{\"blockPath\":[],\"dimensions\":[1],\"domain\":\"\",\"hasChildren\":true,\"lineColor\":\"#77ac30\",\"lineWidth\":2,\"parentID\":1,\"port\":1,\"sid\":[\"\"],\"signalID\":20,\"signalName\":\"signal5\"},\"type\":\"RecordBlkView.Signal\",\"uuid\":\"\"},{\"content\":{\"blockPath\":[],\"dimensions\":[1],\"domain\":\"\",\"leafPath\":\"Bus\\nCreator.signal5.R12\",\"lineColor\":\"#7e2f8e\",\"lineWidth\":2,\"parentID\":20,\"plots\":[ 17 ],\"port\":1,\"sid\":[\"\"],\"signalID\":21,\"signalName\":\"Bus\\nCreator.signal5.R12\"},\"type\":\"RecordBlkView.Signal\",\"uuid\":\"\"},{\"content\":{\"blockPath\":[],\"dimensions\":[1],\"domain\":\"\",\"leafPath\":\"Bus\\nCreator.signal5.R9\",\"lineColor\":\"#77ac30\",\"lineWidth\":2,\"parentID\":20,\"plots\":[ 17 ],\"port\":1,\"sid\":[\"\"],\"signalID\":22,\"signalName\":\"Bus\\nCreator.signal5.R9\"},\"type\":\"RecordBlkView.Signal\",\"uuid\":\"\"},{\"content\":{\"blockPath\":[],\"dimensions\":[1],\"domain\":\"\",\"leafPath\":\"Bus\\nCreator.signal5.R13\",\"lineColor\":\"#4dbeee\",\"lineWidth\":2,\"parentID\":20,\"plots\":[ 17 ],\"port\":1,\"sid\":[\"\"],\"signalID\":23,\"signalName\":\"Bus\\nCreator.signal5.R13\"},\"type\":\"RecordBlkView.Signal\",\"uuid\":\"\"},{\"content\":{\"blockPath\":[],\"dimensions\":[1],\"domain\":\"\",\"leafPath\":\"Bus\\nCreator.signal5.R14\",\"lineColor\":\"#a2142f\",\"lineWidth\":2,\"parentID\":20,\"plots\":[ 17 ],\"port\":1,\"sid\":[\"\"],\"signalID\":24,\"signalName\":\"Bus\\nCreator.signal5.R14\"},\"type\":\"RecordBlkView.Signal\",\"uuid\":\"\"},{\"content\":{\"blockPath\":[],\"dimensions\":[1],\"domain\":\"\",\"hasChildren\":true,\"lineColor\":\"#b746ff\",\"lineWidth\":2,\"parentID\":1,\"port\":1,\"sid\":[\"\"],\"signalID\":25,\"signalName\":\"signal6\"},\"type\":\"RecordBlkView.Signal\",\"uuid\":\"\"},{\"content\":{\"blockPath\":[],\"dimensions\":[1],\"domain\":\"\",\"leafPath\":\"Bus\\nCreator.signal6.R15\",\"lineColor\":\"#ff6929\",\"lineWidth\":2,\"parentID\":25,\"plots\":[ 18 ],\"port\":1,\"sid\":[\"\"],\"signalID\":26,\"signalName\":\"Bus\\nCreator.signal6.R15\"},\"type\":\"RecordBlkView.Signal\",\"uuid\":\"\"},{\"content\":{\"blockPath\":[],\"dimensions\":[1],\"domain\":\"\",\"leafPath\":\"Bus\\nCreator.signal6.R14\",\"lineColor\":\"#b746ff\",\"lineWidth\":2,\"parentID\":25,\"plots\":[ 18 ],\"port\":1,\"sid\":[\"\"],\"signalID\":27,\"signalName\":\"Bus\\nCreator.signal6.R14\"},\"type\":\"RecordBlkView.Signal\",\"uuid\":\"\"},{\"content\":{\"blockPath\":[],\"dimensions\":[1],\"domain\":\"\",\"leafPath\":\"Bus\\nCreator.signal6.R16\",\"lineColor\":\"#64d413\",\"lineWidth\":2,\"parentID\":25,\"plots\":[ 18 ],\"port\":1,\"sid\":[\"\"],\"signalID\":28,\"signalName\":\"Bus\\nCreator.signal6.R16\"},\"type\":\"RecordBlkView.Signal\",\"uuid\":\"\"}]},\"type\":\"RecordBlkView.InputSignals\",\"uuid\":\"\"}],\"packageUris\":[\"http:\\/\\/schema.mathworks.com\\/mf0\\/streamout_blocks\\/R2020a\"],\"version\":\"1.0\"}"
  wires:
  Subsystem 6/1 -> Final/1
  Subsystem 3/5 -> Subsystem 2/2, Substation2/3, Substation3/4  "R8"
  Subsystem 3/3 -> Substation3/2  "R6"
  Final/1 -> Subsystem6/3, Subsystem 6/2  "R16"
  Subsystem 3/1 -> Subsystem 5/3
  Subsystem 1/4 -> Valve Plotter/1(V_S3+1)
  Subsystem 5/3 -> Substation3/5, Subsystem 3/2, Substation5/2  "R9"
  Subsystem 6/4 -> Valve Plotter/6(In6)
  Subsystem 5/2 -> Substation5/1, Subsystem 4/2, Substation4/3  "R12"
  Subsystem 5/1 -> Subsystem 6/3
  Subsystem 3/6 -> Valve Plotter/3(In3)
  Subsystem 1/3 -> Substation1/2  "R2"
  Subsystem 2/4 -> Valve Plotter/2(In2)
  Subsystem 3/2 -> Substation3/1, Substation1/3, Subsystem 1/2  "R5"
  Substation2/1 -> Bus Creator/2, Record4/1, All R/2
  Subsystem 5/4 -> Substation5/3  "R13"
  Subsystem 4/2 -> Substation4/1  "R11"
  Substation5/1 -> Bus Creator/5, Record1/1, All R/5
  Subsystem 4/1 -> Subsystem 5/1
  Substation3/1 -> All R/3, Bus Creator/3, Record3/1
  Subsystem 4/4 -> Valve Plotter/4(In4)
  Subsystem 3/4 -> Substation3/3  "R7"
  Subsystem 6/3 -> Substation5/4, Subsystem 5/2, Subsystem6/2  "R14"
  Subsystem 6/2 -> Subsystem6/1  "R15"
  Substation4/1 -> Bus Creator/4, Record2/1, All R/4
  Substation1/1 -> All R/1, Bus Creator/1, Record5/1
  Subsystem 1/1 -> Subsystem 3/1
  Subsystem 2/3 -> Substation2/2  "R4"
  Subsystem 2/2 -> Substation2/1  "R3"
  Subsystem 1/2 -> Substation1/1  "R1"
  Subsystem 4/3 -> Substation4/2  "R10"
  Subsystem 5/5 -> Valve Plotter/5(In5)
  Subsystem 2/1 -> Subsystem 3/5
  Subsystem 1/5 -> Gain/1
  Subsystem 2/5 -> Gain1/1
  Subsystem 3/7 -> Gain2/1
  Subsystem 4/5 -> Gain3/1
  Subsystem 5/6 -> Gain4/1
  Subsystem 6/5 -> Gain6/1
  Final/2 -> Gain5/1
  Gain/1 -> Rains/1
  Gain1/1 -> Rains/2
  Gain2/1 -> Rains/3
  Gain3/1 -> Rains/4
  Gain4/1 -> Rains/5
  Gain5/1 -> Rains/7
  Gain6/1 -> Rains/6
  Bus Creator/1 -> recordAll/1
  Subsystem6/1 -> Bus Creator/6, Record/1, All R/6
  Subsystem 1/6 -> Spillage calc/1(1), Calculate Total system spillage/1(In1)
  Subsystem 2/6 -> Calculate Total system spillage/2(In2), Spillage calc/2(2)
  Subsystem 3/8 -> Calculate Total system spillage/3(In3), Spillage calc/3(3)
  Subsystem 6/6 -> Spillage calc/6(6), Calculate Total system spillage/6(In6)
  Subsystem 4/6 -> Calculate Total system spillage/4(In4), Spillage calc/4(4)
  Final/3 -> Spillage calc/7(7), Calculate Total system spillage/7(In7)
  Subsystem 5/7 -> Calculate Total system spillage/5(In5), Spillage calc/5(5)
  Calculate Total system spillage/1(Total Spillage) -> Total System spillage/1

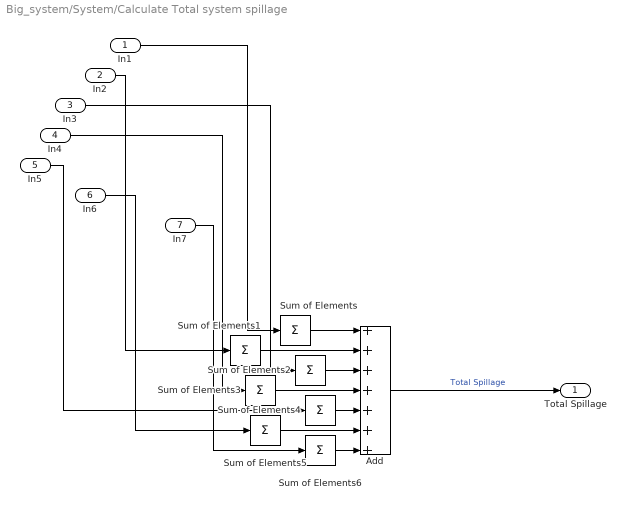
== system Big_system/System/Calculate Total system spillage ==
  In1 : Inport
  In2 : Inport  Port=2
  In3 : Inport  Port=3
  In4 : Inport  Port=4
  In5 : Inport  Port=5
  In6 : Inport  Port=6
  In7 : Inport  Port=7
  Add : Sum  Inputs=+++++++
  Sum of Elements{,1..6} (7 alike) : Sum  Inputs=+
  Total Spillage : Outport
  wires:
  In5/1 -> Sum of Elements4/1
  Sum of Elements4/1 -> Add/5
  Sum of Elements3/1 -> Add/4
  Sum of Elements6/1 -> Add/7
  Sum of Elements2/1 -> Add/3
  Sum of Elements1/1 -> Add/2
  Sum of Elements/1 -> Add/1
  Sum of Elements5/1 -> Add/6
  In2/1 -> Sum of Elements1/1
  In7/1 -> Sum of Elements6/1
  Add/1 -> Total Spillage/1  "Total Spillage"
  In3/1 -> Sum of Elements2/1
  In1/1 -> Sum of Elements/1
  In4/1 -> Sum of Elements3/1
  In6/1 -> Sum of Elements5/1

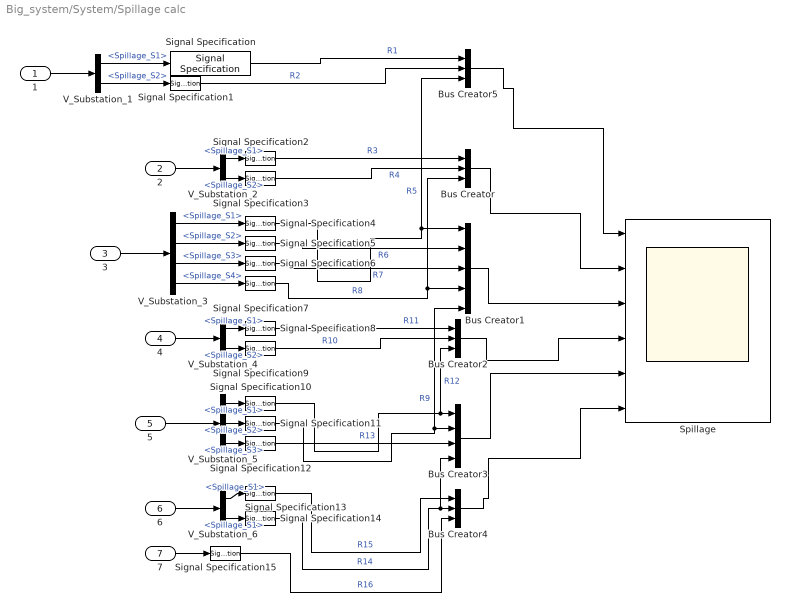
== system Big_system/System/Spillage calc ==
  1 : Inport
  2 : Inport  Port=2
  3 : Inport  Port=3
  4 : Inport  Port=4
  5 : Inport  Port=5
  6 : Inport  Port=6
  7 : Inport  Port=7
  Bus Creator{,2,4..5} (4 alike) : BusCreator  Inputs=3
  Bus Creator1 : BusCreator  Inputs=5
  Bus Creator3 : BusCreator  Inputs=4
  Signal Specification{,1..15} (16 alike) : SignalSpecification
  Spillage : Scope  NumInputPorts=6
      settings: ActiveDisplayString=6  Title=Subsystem 6  ActiveDisplayYMinimum=-1  ActiveDisplayYMaximum=12  YLabel=Total spillage (liters)  DataLoggingVariableName=ScopeData26
  V_Substation_1 : BusSelector  OutputSignals=Spillage_S1,Spillage_S2
  V_Substation_2 : BusSelector  OutputSignals=Spillage_S1,Spillage_S2
  V_Substation_3 : BusSelector  OutputSignals=Spillage_S1,Spillage_S2,Spillage_S3,Spillage_S4
  V_Substation_4 : BusSelector  OutputSignals=Spillage_S1,Spillage_S2
  V_Substation_5 : BusSelector  OutputSignals=Spillage_S1,Spillage_S2,Spillage_S3
  V_Substation_6 : BusSelector  OutputSignals=Spillage_S1,Spillage_S1
  wires:
  1/1 -> V_Substation_1/1
  6/1 -> V_Substation_6/1
  5/1 -> V_Substation_5/1
  4/1 -> V_Substation_4/1
  3/1 -> V_Substation_3/1
  2/1 -> V_Substation_2/1
  Bus Creator5/1 -> Spillage/1
  Bus Creator/1 -> Spillage/2
  Bus Creator2/1 -> Spillage/4
  Bus Creator3/1 -> Spillage/5
  Bus Creator1/1 -> Spillage/3
  V_Substation_6/1 -> Signal Specification13/1  "<Spillage_S1>"
  Bus Creator4/1 -> Spillage/6
  7/1 -> Signal Specification15/1
  V_Substation_6/2 -> Signal Specification14/1  "<Spillage_S1>"
  V_Substation_1/1 -> Signal Specification/1  "<Spillage_S1>"
  V_Substation_1/2 -> Signal Specification1/1  "<Spillage_S2>"
  V_Substation_2/1 -> Signal Specification2/1  "<Spillage_S1>"
  V_Substation_2/2 -> Signal Specification3/1  "<Spillage_S2>"
  V_Substation_3/1 -> Signal Specification4/1  "<Spillage_S1>"
  V_Substation_3/2 -> Signal Specification5/1  "<Spillage_S2>"
  V_Substation_3/3 -> Signal Specification6/1  "<Spillage_S3>"
  V_Substation_3/4 -> Signal Specification7/1  "<Spillage_S4>"
  V_Substation_4/1 -> Signal Specification8/1  "<Spillage_S1>"
  V_Substation_4/2 -> Signal Specification9/1  "<Spillage_S2>"
  V_Substation_5/1 -> Signal Specification10/1  "<Spillage_S1>"
  V_Substation_5/2 -> Signal Specification11/1  "<Spillage_S2>"
  V_Substation_5/3 -> Signal Specification12/1  "<Spillage_S3>"
  Signal Specification1/1 -> Bus Creator5/2  "R2"
  Signal Specification/1 -> Bus Creator5/1  "R1"
  Signal Specification3/1 -> Bus Creator/2  "R4"
  Signal Specification2/1 -> Bus Creator/1  "R3"
  Signal Specification7/1 -> Bus Creator/3, Bus Creator1/4  "R8"
  Signal Specification6/1 -> Bus Creator1/3  "R7"
  Signal Specification5/1 -> Bus Creator1/2  "R6"
  Signal Specification4/1 -> Bus Creator5/3, Bus Creator1/1  "R5"
  Signal Specification9/1 -> Bus Creator2/2  "R10"
  Signal Specification8/1 -> Bus Creator2/1  "R11"
  Signal Specification12/1 -> Bus Creator3/3  "R13"
  Signal Specification11/1 -> Bus Creator1/5, Bus Creator3/2  "R9"
  Signal Specification10/1 -> Bus Creator2/3, Bus Creator3/1  "R12"
  Signal Specification15/1 -> Bus Creator4/3  "R16"
  Signal Specification14/1 -> Bus Creator3/4, Bus Creator4/2  "R14"
  Signal Specification13/1 -> Bus Creator4/1  "R15"

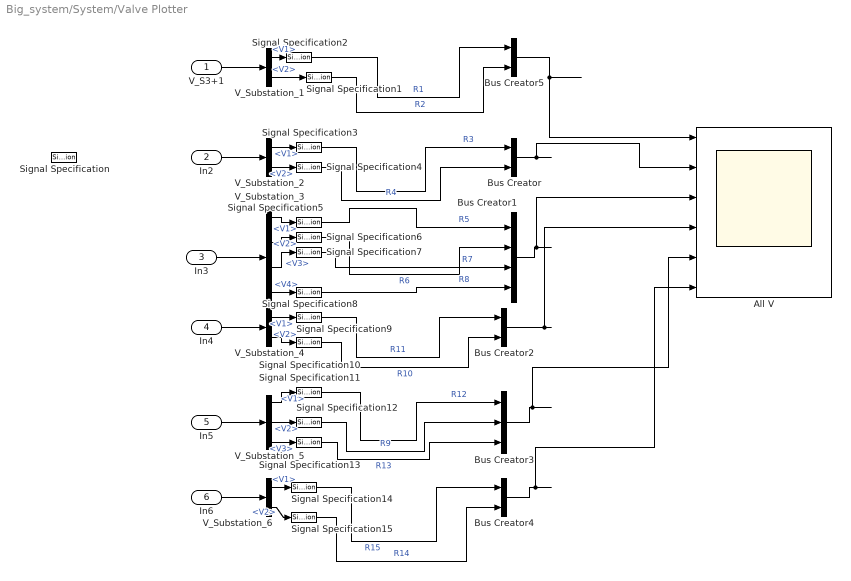
== system Big_system/System/Valve Plotter ==
  V_S3+1 : Inport
  In2 : Inport  Port=2
  In3 : Inport  Port=3
  In4 : Inport  Port=4
  In5 : Inport  Port=5
  In6 : Inport  Port=6
  All V : Scope  NumInputPorts=6
      settings: ActiveDisplayString=6  Title=Subsystem 6  ActiveDisplayYMinimum=-5  ActiveDisplayYMaximum=105  YLabel=Valve opening (%)  DataLoggingVariableName=ScopeData24
  Bus Creator{,2,4..5} (4 alike) : BusCreator  Inputs=2
  Bus Creator1 : BusCreator  Inputs=4
  Bus Creator3 : BusCreator  Inputs=3
  Signal Specification{,1..15} (16 alike) : SignalSpecification
  V_Substation_{1..2,4,6} (4 alike) : BusSelector  OutputSignals=V1,V2
  V_Substation_3 : BusSelector  OutputSignals=V1,V2,V3,V4
  V_Substation_5 : BusSelector  OutputSignals=V1,V2,V3
  wires:
  V_S3+1/1 -> V_Substation_1/1
  In6/1 -> V_Substation_6/1
  In5/1 -> V_Substation_5/1
  In4/1 -> V_Substation_4/1
  In3/1 -> V_Substation_3/1
  In2/1 -> V_Substation_2/1
  V_Substation_1/2 -> Signal Specification1/1  "<V2>"
  Bus Creator5/1 -> All V/1
  Bus Creator/1 -> All V/2
  V_Substation_2/1 -> Signal Specification3/1  "<V1>"
  V_Substation_2/2 -> Signal Specification4/1  "<V2>"
  V_Substation_3/1 -> Signal Specification5/1  "<V1>"
  V_Substation_3/2 -> Signal Specification6/1  "<V2>"
  V_Substation_3/3 -> Signal Specification7/1  "<V3>"
  V_Substation_3/4 -> Signal Specification8/1  "<V4>"
  V_Substation_4/1 -> Signal Specification9/1  "<V1>"
  V_Substation_4/2 -> Signal Specification10/1  "<V2>"
  Bus Creator2/1 -> All V/4
  Bus Creator3/1 -> All V/5
  Bus Creator1/1 -> All V/3
  V_Substation_5/1 -> Signal Specification11/1  "<V1>"
  V_Substation_5/2 -> Signal Specification12/1  "<V2>"
  V_Substation_5/3 -> Signal Specification13/1  "<V3>"
  V_Substation_6/1 -> Signal Specification14/1  "<V1>"
  V_Substation_6/2 -> Signal Specification15/1  "<V2>"
  Bus Creator4/1 -> All V/6
  V_Substation_1/1 -> Signal Specification2/1  "<V1>"
  Signal Specification1/1 -> Bus Creator5/2  "R2"
  Signal Specification2/1 -> Bus Creator5/1  "R1"
  Signal Specification4/1 -> Bus Creator/2  "R4"
  Signal Specification3/1 -> Bus Creator/1  "R3"
  Signal Specification8/1 -> Bus Creator1/4  "R8"
  Signal Specification7/1 -> Bus Creator1/3  "R7"
  Signal Specification6/1 -> Bus Creator1/2  "R6"
  Signal Specification5/1 -> Bus Creator1/1  "R5"
  Signal Specification10/1 -> Bus Creator2/2  "R10"
  Signal Specification9/1 -> Bus Creator2/1  "R11"
  Signal Specification13/1 -> Bus Creator3/3  "R13"
  Signal Specification12/1 -> Bus Creator3/2  "R9"
  Signal Specification11/1 -> Bus Creator3/1  "R12"
  Signal Specification15/1 -> Bus Creator4/2  "R14"
  Signal Specification14/1 -> Bus Creator4/1  "R15"
